simulink model "hydraulicsys"  (R2020b)
settings: Solver=FixedStepAuto  StartTime=0.0  StopTime=90  FixedStep=0.01  RelTol=1e-3
InitFcn:
  | config_presse
values from neighbouring files (symbols this model uses):
  G_s = 0.15    [config_presse.m]
  t_09 = 15    [config_presse.m]
  T_max = 90    [config_presse.m]
  T_min = -40    [config_presse.m]
settings Model: EnablePacing=on  Creator=mateu  LastModifiedBy=mateu

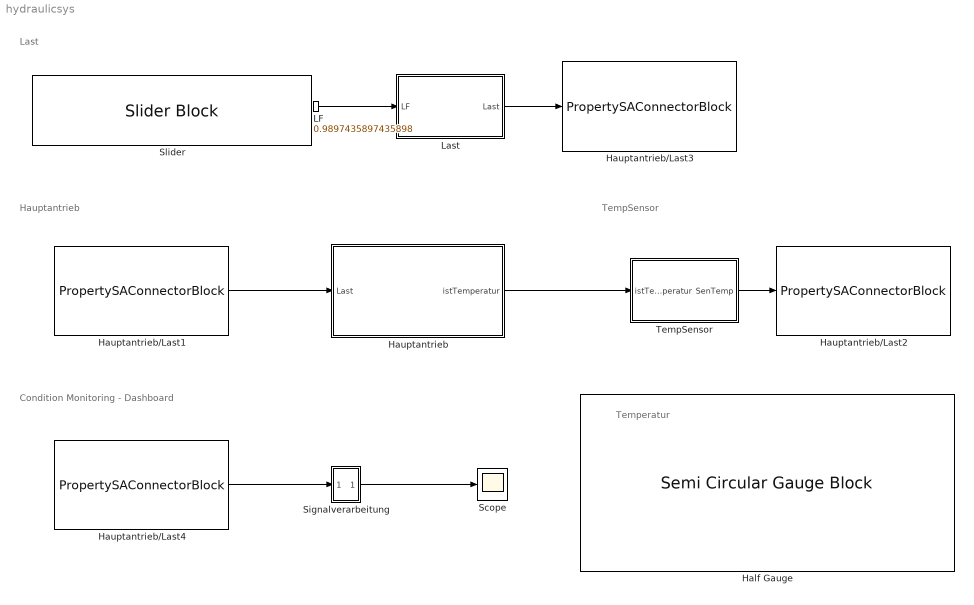
== system hydraulicsys ==
  note: Temperatur
  note: TempSensor
  note: Last
  note: Hauptantrieb
  note: Condition Monitoring - Dashboard
  Half Gauge : SemiCircularGaugeBlock  LabelPosition=Hide  ScaleMin=-10
  Hauptantrieb : Subsystem
  Hauptantrieb/Last1 : S-Function  FunctionName=PropertySAConnectorBlock  Parameters=bm, sr, regUrlStr, aasUrlStr, aasId, smId, seId  SFunctionDeploymentMode=off  EnableBusSupport=off  mask{bmStr=Real-time, conMethod=via RegistryServer, aasUrlStr_=http://localhost:4001/aasServer/shells/https%3A%2F%2Fexample.com%2Fids%2Faas%2F6001_2130_8022_6165/aas, regUrlStr=http://localhost:8082/registry/api/v1/registry, sr=0.5, aasId=https://example.com/ids/aas/6001_2130_8022_6165, smId=Hauptantrieb, seId=last, bm=1, aasUrlStr=}
      mask prompts: bmStr "Operation Mode"; conMethod "Connection Method"; aasUrlStr_ "AAS Url"; regUrlStr "Registry URL"; sr "Sample Rate"; aasId "AAS Id"; smId "Submodel IdShort"; seId "Property IdShort"
      mask TypeOptions bmStr: Snapshot | Real-time
      mask Callback bmStr:
      | bmStr = get_param(gcb,'bmStr');
      | vis = get_param(gcb,'MaskVisibilities');
      | 
      | switch bmStr
      |     case 'Snapshot'
      |         set_param(gcb, 'bm', "0");
      |         vis(5) = {'off'};
      |         set_param(gcb, 'MaskVisibilities', vis);
      |     case 'Real-time'
      |         set_param(gcb, 'bm',  "1");
      |         vis(5) = {'on'};
      |         set_param(gcb, 'MaskVisibilities', vis);
      | end
      mask TypeOptions conMethod: via RegistryServer | via AAS URL
      mask Callback conMethod:
      | conMethod = get_param(gcb,'conMethod');
      | aasUrlStr = get_param(gcb,'aasUrlStr_');
      | vis = get_param(gcb,'MaskVisibilities');
      | 
      | switch conMethod
      |     case 'via RegistryServer'
      |         vis(3) = {'off'};
      |         vis(4) = {'on'};
      |         set_param(gcb, 'MaskVisibilities', vis);
      |         set_param(gcb, 'aasUrlStr', '');
      |     case 'via AAS URL'
      |         vis(3) = {'on'};
      |         vis(4) = {'off'};
      |         set_param(gcb, 'MaskVisibilities', vis);
      |         set_param(gcb, 'aasUrlStr', aasUrlStr);
      | end
      mask Callback aasUrlStr_:
      | conMethod = get_param(gcb,'conMethod');
      | aasUrlStr = get_param(gcb,'aasUrlStr_');
      | switch conMethod
      |     case 'via AAS URL'
      |         set_param(gcb, 'aasUrlStr', aasUrlStr);
      | end
      mask DialogControl DescGroupVar Prompt: Standalone Property Block
      mask DialogControl DescTextVar Prompt: This block connects to a SubmodelElement running in an AAS Server. Data sent to the block's input updates the value of the SubmodelElement, whereas its current value is sent to the block's output. This process can be executed in two operation modes: Snapshot mode, wherein the input routine is executed at the beginining and the output routine at the end of the simulation; Real-time mode, by which is assumed that the wall clock is the same as the simulation clock and the input/output routines are executed in the specified sample rate.
      mask Display:
      | bm = get_param(gcb,'bm')
      | sr = get_param(gcb,'sr')
      | aas = replace(get_param(gcb,'aasId'),"_","\_");
      | sm = replace(get_param(gcb,'smId'),"_","\_");
      | se = replace(get_param(gcb,'seId'),"_","\_");
      | 
      | pos = get_param(gcb, 'Position');
      | w = pos(3) - pos(1);
      | h = pos(4) - pos(2);
      | 
      | full = sm  + "/" + se
      | text(5,20, "{\bf\fontsize{7}"+aas+"}", 'texmode','on')
      | text(5,10, "{\bf\fontsize{6}"+full+"}", 'texmode','on')
      | image('basyx.png', [w-15,h-20,10,15]);
      | 
      | if bm=="1"
      |     port_label('output', 1,"{\bf\fontsize{6}sr="+sr+"s}", 'texmode','on')
      | end
  Hauptantrieb/Last2 : S-Function  FunctionName=PropertySAConnectorBlock  Parameters=bm, sr, regUrlStr, aasUrlStr, aasId, smId, seId  SFunctionDeploymentMode=off  EnableBusSupport=off  mask{bmStr=Real-time, conMethod=via RegistryServer, aasUrlStr_=http://localhost:4001/aasServer/shells/https%3A%2F%2Fexample.com%2Fids%2Faas%2F6001_2130_8022_6165/aas, regUrlStr=http://localhost:8082/registry/api/v1/registry, sr=0.1, aasId=https://example.com/ids/aas/6001_2130_8022_6165, smId=TempSensor, seId=temperatur, bm=1, aasUrlStr=}
      mask prompts: bmStr "Operation Mode"; conMethod "Connection Method"; aasUrlStr_ "AAS Url"; regUrlStr "Registry URL"; sr "Sample Rate"; aasId "AAS Id"; smId "Submodel IdShort"; seId "Property IdShort"
      mask TypeOptions bmStr: Snapshot | Real-time
      mask Callback bmStr:
      | bmStr = get_param(gcb,'bmStr');
      | vis = get_param(gcb,'MaskVisibilities');
      | 
      | switch bmStr
      |     case 'Snapshot'
      |         set_param(gcb, 'bm', "0");
      |         vis(5) = {'off'};
      |         set_param(gcb, 'MaskVisibilities', vis);
      |     case 'Real-time'
      |         set_param(gcb, 'bm',  "1");
      |         vis(5) = {'on'};
      |         set_param(gcb, 'MaskVisibilities', vis);
      | end
      mask TypeOptions conMethod: via RegistryServer | via AAS URL
      mask Callback conMethod:
      | conMethod = get_param(gcb,'conMethod');
      | aasUrlStr = get_param(gcb,'aasUrlStr_');
      | vis = get_param(gcb,'MaskVisibilities');
      | 
      | switch conMethod
      |     case 'via RegistryServer'
      |         vis(3) = {'off'};
      |         vis(4) = {'on'};
      |         set_param(gcb, 'MaskVisibilities', vis);
      |         set_param(gcb, 'aasUrlStr', '');
      |     case 'via AAS URL'
      |         vis(3) = {'on'};
      |         vis(4) = {'off'};
      |         set_param(gcb, 'MaskVisibilities', vis);
      |         set_param(gcb, 'aasUrlStr', aasUrlStr);
      | end
      mask Callback aasUrlStr_:
      | conMethod = get_param(gcb,'conMethod');
      | aasUrlStr = get_param(gcb,'aasUrlStr_');
      | switch conMethod
      |     case 'via AAS URL'
      |         set_param(gcb, 'aasUrlStr', aasUrlStr);
      | end
      mask DialogControl DescGroupVar Prompt: Standalone Property Block
      mask DialogControl DescTextVar Prompt: This block connects to a SubmodelElement running in an AAS Server. Data sent to the block's input updates the value of the SubmodelElement, whereas its current value is sent to the block's output. This process can be executed in two operation modes: Snapshot mode, wherein the input routine is executed at the beginining and the output routine at the end of the simulation; Real-time mode, by which is assumed that the wall clock is the same as the simulation clock and the input/output routines are executed in the specified sample rate.
      mask Display:
      | bm = get_param(gcb,'bm')
      | sr = get_param(gcb,'sr')
      | aas = replace(get_param(gcb,'aasId'),"_","\_");
      | sm = replace(get_param(gcb,'smId'),"_","\_");
      | se = replace(get_param(gcb,'seId'),"_","\_");
      | 
      | pos = get_param(gcb, 'Position');
      | w = pos(3) - pos(1);
      | h = pos(4) - pos(2);
      | 
      | full = sm  + "/" + se
      | text(5,20, "{\bf\fontsize{7}"+aas+"}", 'texmode','on')
      | text(5,10, "{\bf\fontsize{6}"+full+"}", 'texmode','on')
      | image('basyx.png', [w-15,h-20,10,15]);
      | 
      | if bm=="1"
      |     port_label('output', 1,"{\bf\fontsize{6}sr="+sr+"s}", 'texmode','on')
      | end
  Hauptantrieb/Last3 : S-Function  FunctionName=PropertySAConnectorBlock  Parameters=bm, sr, regUrlStr, aasUrlStr, aasId, smId, seId  SFunctionDeploymentMode=off  EnableBusSupport=off  mask{bmStr=Real-time, conMethod=via RegistryServer, aasUrlStr_=http://localhost:4001/aasServer/shells/https%3A%2F%2Fexample.com%2Fids%2Faas%2F6001_2130_8022_6165/aas, regUrlStr=http://localhost:8082/registry/api/v1/registry, sr=0.5, aasId=https://example.com/ids/aas/6001_2130_8022_6165, smId=Hauptantrieb, seId=last, bm=1, aasUrlStr=}
      mask prompts: bmStr "Operation Mode"; conMethod "Connection Method"; aasUrlStr_ "AAS Url"; regUrlStr "Registry URL"; sr "Sample Rate"; aasId "AAS Id"; smId "Submodel IdShort"; seId "Property IdShort"
      mask TypeOptions bmStr: Snapshot | Real-time
      mask Callback bmStr:
      | bmStr = get_param(gcb,'bmStr');
      | vis = get_param(gcb,'MaskVisibilities');
      | 
      | switch bmStr
      |     case 'Snapshot'
      |         set_param(gcb, 'bm', "0");
      |         vis(5) = {'off'};
      |         set_param(gcb, 'MaskVisibilities', vis);
      |     case 'Real-time'
      |         set_param(gcb, 'bm',  "1");
      |         vis(5) = {'on'};
      |         set_param(gcb, 'MaskVisibilities', vis);
      | end
      mask TypeOptions conMethod: via RegistryServer | via AAS URL
      mask Callback conMethod:
      | conMethod = get_param(gcb,'conMethod');
      | aasUrlStr = get_param(gcb,'aasUrlStr_');
      | vis = get_param(gcb,'MaskVisibilities');
      | 
      | switch conMethod
      |     case 'via RegistryServer'
      |         vis(3) = {'off'};
      |         vis(4) = {'on'};
      |         set_param(gcb, 'MaskVisibilities', vis);
      |         set_param(gcb, 'aasUrlStr', '');
      |     case 'via AAS URL'
      |         vis(3) = {'on'};
      |         vis(4) = {'off'};
      |         set_param(gcb, 'MaskVisibilities', vis);
      |         set_param(gcb, 'aasUrlStr', aasUrlStr);
      | end
      mask Callback aasUrlStr_:
      | conMethod = get_param(gcb,'conMethod');
      | aasUrlStr = get_param(gcb,'aasUrlStr_');
      | switch conMethod
      |     case 'via AAS URL'
      |         set_param(gcb, 'aasUrlStr', aasUrlStr);
      | end
      mask DialogControl DescGroupVar Prompt: Standalone Property Block
      mask DialogControl DescTextVar Prompt: This block connects to a SubmodelElement running in an AAS Server. Data sent to the block's input updates the value of the SubmodelElement, whereas its current value is sent to the block's output. This process can be executed in two operation modes: Snapshot mode, wherein the input routine is executed at the beginining and the output routine at the end of the simulation; Real-time mode, by which is assumed that the wall clock is the same as the simulation clock and the input/output routines are executed in the specified sample rate.
      mask Display:
      | bm = get_param(gcb,'bm')
      | sr = get_param(gcb,'sr')
      | aas = replace(get_param(gcb,'aasId'),"_","\_");
      | sm = replace(get_param(gcb,'smId'),"_","\_");
      | se = replace(get_param(gcb,'seId'),"_","\_");
      | 
      | pos = get_param(gcb, 'Position');
      | w = pos(3) - pos(1);
      | h = pos(4) - pos(2);
      | 
      | full = sm  + "/" + se
      | text(5,20, "{\bf\fontsize{7}"+aas+"}", 'texmode','on')
      | text(5,10, "{\bf\fontsize{6}"+full+"}", 'texmode','on')
      | image('basyx.png', [w-15,h-20,10,15]);
      | 
      | if bm=="1"
      |     port_label('output', 1,"{\bf\fontsize{6}sr="+sr+"s}", 'texmode','on')
      | end
  Hauptantrieb/Last4 : S-Function  FunctionName=PropertySAConnectorBlock  Parameters=bm, sr, regUrlStr, aasUrlStr, aasId, smId, seId  SFunctionDeploymentMode=off  EnableBusSupport=off  mask{bmStr=Real-time, conMethod=via RegistryServer, aasUrlStr_=http://localhost:4001/aasServer/shells/https%3A%2F%2Fexample.com%2Fids%2Faas%2F6001_2130_8022_6165/aas, regUrlStr=http://localhost:8082/registry/api/v1/registry, sr=0.1, aasId=https://example.com/ids/aas/6001_2130_8022_6165, smId=TempSensor, seId=temperatur, bm=1, aasUrlStr=}
      mask prompts: bmStr "Operation Mode"; conMethod "Connection Method"; aasUrlStr_ "AAS Url"; regUrlStr "Registry URL"; sr "Sample Rate"; aasId "AAS Id"; smId "Submodel IdShort"; seId "Property IdShort"
      mask TypeOptions bmStr: Snapshot | Real-time
      mask Callback bmStr:
      | bmStr = get_param(gcb,'bmStr');
      | vis = get_param(gcb,'MaskVisibilities');
      | 
      | switch bmStr
      |     case 'Snapshot'
      |         set_param(gcb, 'bm', "0");
      |         vis(5) = {'off'};
      |         set_param(gcb, 'MaskVisibilities', vis);
      |     case 'Real-time'
      |         set_param(gcb, 'bm',  "1");
      |         vis(5) = {'on'};
      |         set_param(gcb, 'MaskVisibilities', vis);
      | end
      mask TypeOptions conMethod: via RegistryServer | via AAS URL
      mask Callback conMethod:
      | conMethod = get_param(gcb,'conMethod');
      | aasUrlStr = get_param(gcb,'aasUrlStr_');
      | vis = get_param(gcb,'MaskVisibilities');
      | 
      | switch conMethod
      |     case 'via RegistryServer'
      |         vis(3) = {'off'};
      |         vis(4) = {'on'};
      |         set_param(gcb, 'MaskVisibilities', vis);
      |         set_param(gcb, 'aasUrlStr', '');
      |     case 'via AAS URL'
      |         vis(3) = {'on'};
      |         vis(4) = {'off'};
      |         set_param(gcb, 'MaskVisibilities', vis);
      |         set_param(gcb, 'aasUrlStr', aasUrlStr);
      | end
      mask Callback aasUrlStr_:
      | conMethod = get_param(gcb,'conMethod');
      | aasUrlStr = get_param(gcb,'aasUrlStr_');
      | switch conMethod
      |     case 'via AAS URL'
      |         set_param(gcb, 'aasUrlStr', aasUrlStr);
      | end
      mask DialogControl DescGroupVar Prompt: Standalone Property Block
      mask DialogControl DescTextVar Prompt: This block connects to a SubmodelElement running in an AAS Server. Data sent to the block's input updates the value of the SubmodelElement, whereas its current value is sent to the block's output. This process can be executed in two operation modes: Snapshot mode, wherein the input routine is executed at the beginining and the output routine at the end of the simulation; Real-time mode, by which is assumed that the wall clock is the same as the simulation clock and the input/output routines are executed in the specified sample rate.
      mask Display:
      | bm = get_param(gcb,'bm')
      | sr = get_param(gcb,'sr')
      | aas = replace(get_param(gcb,'aasId'),"_","\_");
      | sm = replace(get_param(gcb,'smId'),"_","\_");
      | se = replace(get_param(gcb,'seId'),"_","\_");
      | 
      | pos = get_param(gcb, 'Position');
      | w = pos(3) - pos(1);
      | h = pos(4) - pos(2);
      | 
      | full = sm  + "/" + se
      | text(5,20, "{\bf\fontsize{7}"+aas+"}", 'texmode','on')
      | text(5,10, "{\bf\fontsize{6}"+full+"}", 'texmode','on')
      | image('basyx.png', [w-15,h-20,10,15]);
      | 
      | if bm=="1"
      |     port_label('output', 1,"{\bf\fontsize{6}sr="+sr+"s}", 'texmode','on')
      | end
  LF : Constant  Value=0.9897435897435898
  Last : Subsystem
  Scope : Scope
  Signalverarbeitung : Subsystem
  Slider : SliderBlock  ScaleMax=1  TickInterval=0.1
  TempSensor : Subsystem
  wires:
  Hauptantrieb/Last1/1 -> Hauptantrieb/1(Last)
  Hauptantrieb/Last4/1 -> Signalverarbeitung/1(In1)
  Signalverarbeitung/1(Out1) -> Scope/1
  LF/1 -> Last/1(LF)
  Hauptantrieb/1(istTemperatur) -> TempSensor/1(istTemperatur)
  TempSensor/1(SenTemp) -> Hauptantrieb/Last2/1
  Last/1(Last) -> Hauptantrieb/Last3/1

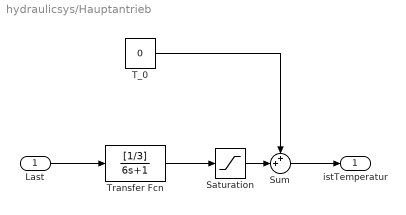
== system hydraulicsys/Hauptantrieb ==
  Last : Inport
  Saturation : Saturate  UpperLimit=150  LowerLimit=0
  Sum : Sum  Inputs=++|
  T_0 : Constant  Value=0
  Transfer Fcn : TransferFcn  Numerator=[1/3]  Denominator=[6 1]
  istTemperatur : Outport
  wires:
  Last/1 -> Transfer Fcn/1
  T_0/1 -> Sum/1
  Sum/1 -> istTemperatur/1
  Transfer Fcn/1 -> Saturation/1
  Saturation/1 -> Sum/2

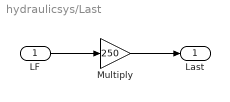
== system hydraulicsys/Last ==
  LF : Inport
  Multiply : Gain  Gain=250
  Last : Outport
  wires:
  Multiply/1 -> Last/1
  LF/1 -> Multiply/1

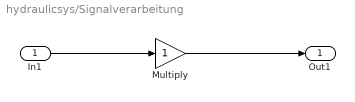
== system hydraulicsys/Signalverarbeitung ==
  In1 : Inport
  Multiply : Gain
  Out1 : Outport
  wires:
  Multiply/1 -> Out1/1
  In1/1 -> Multiply/1

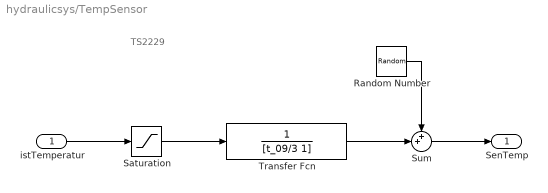
== system hydraulicsys/TempSensor ==
  note: TS2229
  istTemperatur : Inport
  Random Number : RandomNumber  Variance=G_s/32  Seed=202021
  Saturation : Saturate  UpperLimit=T_max  LowerLimit=T_min
  Sum : Sum  Inputs=++|
  Transfer Fcn : TransferFcn  Denominator=[t_09/3 1]
  SenTemp : Outport
  wires:
  Transfer Fcn/1 -> Sum/2
  Saturation/1 -> Transfer Fcn/1
  Sum/1 -> SenTemp/1
  istTemperatur/1 -> Saturation/1
  Random Number/1 -> Sum/1
